simulink model "Practica1"  (R2025b)
settings: Solver=VariableStepAuto  StartTime=0.0  StopTime=200  RelTol=1e-3  AbsTol=1e-3
undefined symbols (not defined in the file): J, Km, L_a, R_a
libraries: fl_lib x13, nesl_utility x8
settings Model: Creator=chenfu  LastModifiedBy=chenfu
settings SolverCC: AutoScaleAbsTol=off  AlgebraicLoopSolver=TrustRegion  MaxZcPerStep=1.0
settings DebuggingCC: UnconnectedInputMsg=warning  UnconnectedOutputMsg=warning  UnconnectedLineMsg=warning  SymbolicDimsDataTypeCodeGenerationDiagnostic=none
settings ModelReferenceCC: EnableRefExpFcnMdlSchedulingChecks=on
settings SFSimCC: CustomCodeUndefinedFunction=UseInterfaceOnly
settings RTWCC: GPUComputeCapability=3.5  DLArmComputeVersion=19.05
settings SimscapeCC: SimscapeLogType=all  SimscapeLogSimulationStatistics=on  SimscapeLogDataHistory=10000.0

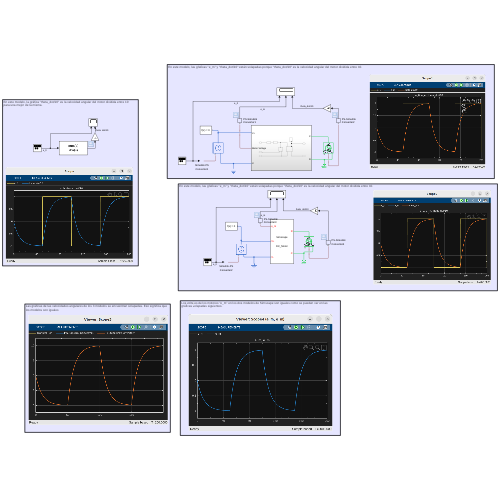
[thumbnail: Simulink's stored preview of the top-level diagram]
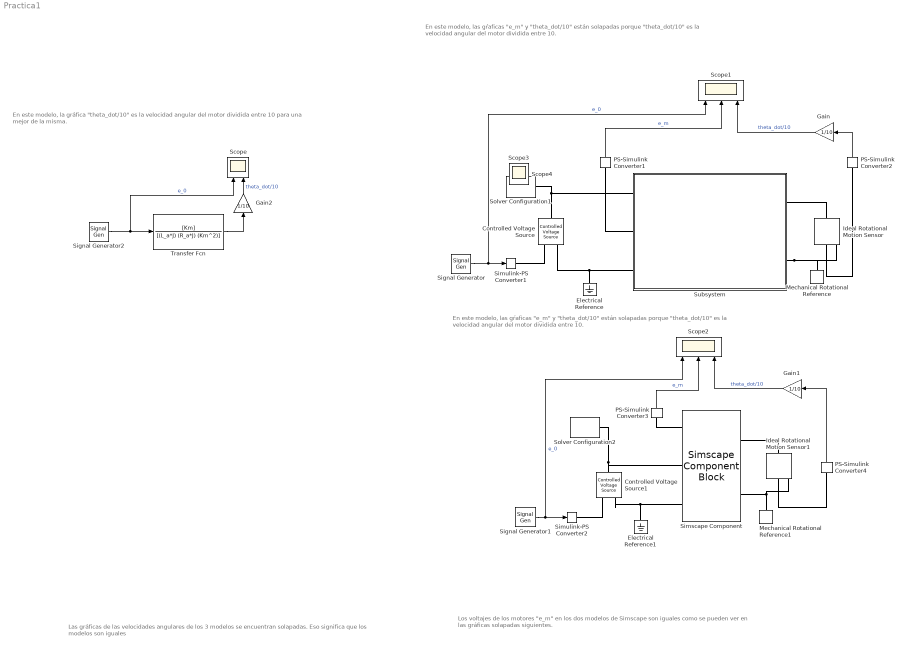
== system Practica1 ==
  note: En este modelo, la gráfica "theta_dot/10" es la velocidad angular del motor dividida entre 10
      | para una mejor de la misma.
  note: En este modelo, las gŕaficas "e_m" y "theta_dot/10" están solapadas porque "theta_dot/10" es la velocidad angular del motor dividida entre 10.
  note: En este modelo, las gŕaficas "e_m" y "theta_dot/10" están solapadas porque "theta_dot/10" es la velocidad angular del motor dividida entre 10.
  note: Los voltajes de los motores "e_m" en los dos modelos de Simscape son iguales como se pueden ver en las
      | gráficas solapadas siguientes.
  note: Las gráficas de las velocidades angulares de los 3 modelos se encuentran solapadas. Eso significa que
      | los modelos son iguales
  Controlled Voltage Source : fl_lib/Electrical/Electrical Sources/Controlled Voltage Source
  Controlled Voltage Source1 : fl_lib/Electrical/Electrical Sources/Controlled Voltage Source
  Electrical Reference : fl_lib/Electrical/Electrical Elements/Electrical Reference
  Electrical Reference1 : fl_lib/Electrical/Electrical Elements/Electrical Reference
  Gain : Gain  Gain=1/10
  Gain1 : Gain  Gain=1/10
  Gain2 : Gain  Gain=1/10
  Ideal Rotational Motion Sensor : fl_lib/Mechanical/Mechanical Sensors/Ideal Rotational Motion Sensor  reference=foundation.enum.MeasurementReference.difference  acceleration_port=false  velocity_port=true  position_port=true  wrap_angle=false  offset=0 rad
  Ideal Rotational Motion Sensor1 : fl_lib/Mechanical/Mechanical Sensors/Ideal Rotational Motion Sensor  reference=foundation.enum.MeasurementReference.difference  acceleration_port=false  velocity_port=true  position_port=true  wrap_angle=false  offset=0 rad
  Mechanical Rotational Reference : fl_lib/Mechanical/Rotational Elements/Mechanical Rotational Reference
  Mechanical Rotational Reference1 : fl_lib/Mechanical/Rotational Elements/Mechanical Rotational Reference
  PS-Simulink Converter{1..4} (4 alike) : nesl_utility/PS-Simulink Converter  PhysicalDomain=network_engine_domain  SubClassName=ps_output  LeftPortType=input  RightPortType=output  PseudoPeriodic=off  Frequencies=[]  VectorFormat=inherit  Unit=inherit  AffineConversion=off
  Scope : Scope  NumInputPorts=2
      settings: ActiveDisplayYMinimum=-1.25  ActiveDisplayYMaximum=1.25  DataLoggingVariableName=ScopeData2
  Scope1 : Scope  NumInputPorts=3
      settings: ActiveDisplayYMinimum=-1  ActiveDisplayYMaximum=1
  Scope2 : Scope  NumInputPorts=3
      settings: ActiveDisplayYMinimum=-1.25  ActiveDisplayYMaximum=1.25
  Signal Generator : SignalGenerator  WaveForm=square  Frequency=0.01
  Signal Generator1 : SignalGenerator  WaveForm=square  Frequency=0.01
  Signal Generator2 : SignalGenerator  WaveForm=square  Frequency=0.01
  Simscape Component : SimscapeComponentBlock  SourceFile=DC_Motor  ComponentPath=DC_Motor  ComponentVariants="[\"DC_Motor\"]"  ComponentVariantNames="[\"DC_Motor\"]"  ClassName=DC_Motor  SchemaVersion=1  res=10.0 Ohm  l=1e-2 H  J=1e-2 kg*m^2  bEMF=1e-1 V*s/rad  e_o_specify=off  e_o_priority=None  e_o=0 V  e_o_nominal_specify=off  e_o_nominal_value=1  e_o_nominal_unit=V  e_m_specify=off  e_m_priority=None  e_m=0 V  e_m_nominal_specify=off  e_m_nominal_value=1  e_m_nominal_unit=V  w_specify=off  w_priority=None  w=0 rad/s  w_nominal_specify=off  w_nominal_value=1  w_nominal_unit=rad/s  t_specify=off  t_priority=None  t=0 N*m  t_nominal_specify=off  t_nominal_value=1  t_nominal_unit=N*m  i_specify=off  i_priority=None  i=0 A  i_nominal_specify=off  i_nominal_value=1  i_nominal_unit=A
      settings: CopyFcn=simscape.sscblock.internal.componentBlockCallback(gcbh,'COPY')  PreCopyFcn=simscape.sscblock.internal.componentBlockCallback(gcbh,'PRECOPY')  PreDeleteFcn=simscape.sscblock.internal.componentBlockCallback(gcbh,'PREDELETE')  InternalSimscapePortConfiguration="{\"Bottom\":[],\"Left\":[{\"id\":\"V\",\"label\":\"e_m\",\"type\":\"output\"},{\"id\":\"vmas\",\"label\":\"V+\",\"type\":\"foundation.electrical.electrical\"},{\"id\":\"vmenos\",\"label\":\"V-\",\"type\":\"foundation.electrical.electrical\"}],\"Right\":[{\"id\":\"R\",\"label\":\"R\",\"type\":\"foundation.mechanical.rotational.rotational\"},{\"id\":\"C\",\"label\":\"C\",\"type\":\"foundation.mechanical.rotational.rotational\"}],\"Top\":[]}"
      mask Type: Simple Simscape component
  Simulink-PS Converter1 : nesl_utility/Simulink-PS Converter  PhysicalDomain=network_engine_domain  SubClassName=ps_input  LeftPortType=input  RightPortType=output  PseudoPeriodic=off  Frequencies=[]  NoiseDistribution=none  NoiseParameters=[]  Unit=1  AffineConversion=off  FilteringAndDerivatives=provide  SimscapeFilterOrder=1  InputFilterTimeConstant=0.001  UdotUserProvided=0
  Simulink-PS Converter2 : nesl_utility/Simulink-PS Converter  PhysicalDomain=network_engine_domain  SubClassName=ps_input  LeftPortType=input  RightPortType=output  PseudoPeriodic=off  Frequencies=[]  NoiseDistribution=none  NoiseParameters=[]  Unit=1  AffineConversion=off  FilteringAndDerivatives=filter  SimscapeFilterOrder=1  InputFilterTimeConstant=0.001  UdotUserProvided=0
  Solver Configuration1 : nesl_utility/Solver Configuration  PhysicalDomain=network_engine_domain  SubClassName=solver  LeftPortType=input  RightPortType=generic  Tones=[]  Harmonics=[]  SimulateNoise=off  Profile=off  UseLocalSampling=off  EnableSwitchedLinearOptims=on  FrequencyDomain=off  UseCCode=off  RelTol=0.001  AbsTol=0.001  MinStep=1e-09  ToWorkspace=off  RevertToSquareIcSolve=off  NumHomotopyIterations=100  PhasorMode=off  PhasorModeNumHarmonics=1  ConsistencySolver=NEWTON_XTOL_AFTER_FTOL  IndexReductionMethod=DerivativeReplacement  DoDC=off  ResidualTolerance=1e-09  ConsistencyTolSource=GLOBAL  ConsistencyAbsTol=0.001  ConsistencyRelTol=0.001  ConsistencyTolFactor=0.001  UseLocalSolver=off  LocalSolverChoice=NE_BACKWARD_EULER_ADVANCER  ResolveIndetEquations=on  FunctionEvalNumThread=1  LocalSolverSampleTime=0.001  DoFixedCost=off  MaxNonlinIter=3  MaxModeIter=2  ComputeImpulses=off  ImpulseIterations=2  LinearAlgebra=auto  LinearAlgebraNumThread=0  EquationFormulation=NE_TIME_EF  DelaysMemoryBudget=1024  AutomaticFiltering=on  FilteringTimeConstant=0.001  PartitionStorageMethod=AS_NEEDED  PartitionMemoryBudget=1024  PartitionMethod=ROBUST  MultibodyUseLocalSolver=off  MultibodyLocalSolverChoice=ODE1  MultibodyLocalSolverSampleTime=0.001
  Solver Configuration2 : nesl_utility/Solver Configuration  PhysicalDomain=network_engine_domain  SubClassName=solver  LeftPortType=input  RightPortType=generic  Tones=[]  Harmonics=[]  SimulateNoise=off  Profile=off  UseLocalSampling=off  EnableSwitchedLinearOptims=on  FrequencyDomain=off  UseCCode=off  RelTol=0.001  AbsTol=0.001  MinStep=1e-09  ToWorkspace=off  RevertToSquareIcSolve=off  NumHomotopyIterations=100  PhasorMode=off  PhasorModeNumHarmonics=1  ConsistencySolver=NEWTON_XTOL_AFTER_FTOL  IndexReductionMethod=DerivativeReplacement  DoDC=off  ResidualTolerance=1e-09  ConsistencyTolSource=GLOBAL  ConsistencyAbsTol=0.001  ConsistencyRelTol=0.001  ConsistencyTolFactor=0.001  UseLocalSolver=off  LocalSolverChoice=NE_BACKWARD_EULER_ADVANCER  ResolveIndetEquations=on  FunctionEvalNumThread=1  LocalSolverSampleTime=0.001  DoFixedCost=off  MaxNonlinIter=3  MaxModeIter=2  ComputeImpulses=off  ImpulseIterations=2  LinearAlgebra=auto  LinearAlgebraNumThread=0  EquationFormulation=NE_TIME_EF  DelaysMemoryBudget=1024  AutomaticFiltering=on  FilteringTimeConstant=0.001  PartitionStorageMethod=AS_NEEDED  PartitionMemoryBudget=1024  PartitionMethod=ROBUST  MultibodyUseLocalSolver=off  MultibodyLocalSolverChoice=ODE1  MultibodyLocalSolverSampleTime=0.001
  Subsystem : Subsystem
  Transfer Fcn : TransferFcn  Numerator=[Km]  Denominator=[(L_a*J) (R_a*J) (Km^2)]
  Scope3 : Scope
      settings: ActiveDisplayYMinimum=-12.405916089896222  ActiveDisplayYMaximum=12.338623681139223  DataLoggingVariableName=ScopeData3
  Scope4 : Scope
      settings: ActiveDisplayYMinimum=-1.2405916089222164  ActiveDisplayYMaximum=1.2338623675072702  DataLoggingVariableName=ScopeData4
  wires:
  Signal Generator/1 -> Scope1/1, Simulink-PS Converter1/1  "e_0"
  PS-Simulink Converter1/1 -> Scope1/2  "e_m"
  Gain/1 -> Scope1/3  "theta_dot/10"
  PS-Simulink Converter2/1 -> Gain/1
  Signal Generator1/1 -> Scope2/1, Simulink-PS Converter2/1  "e_0"
  PS-Simulink Converter4/1 -> Gain1/1
  PS-Simulink Converter3/1 -> Scope2/2  "e_m"
  Signal Generator2/1 -> Scope/1, Transfer Fcn/1  "e_0"
  Transfer Fcn/1 -> Gain2/1
  Gain2/1 -> Scope/2  "theta_dot/10"
  Gain1/1 -> Scope2/3  "theta_dot/10"
  connections:
  Controlled Voltage Source/LConn1 -- Solver Configuration1/RConn1 -- Subsystem/LConn1
  Controlled Voltage Source/RConn2 -- Electrical Reference/LConn1 -- Subsystem/LConn3
  Simulink-PS Converter1/RConn1 -- Controlled Voltage Source/RConn1
  Subsystem/RConn1 -- Ideal Rotational Motion Sensor/LConn1
  Subsystem/RConn2 -- Ideal Rotational Motion Sensor/RConn1 -- Mechanical Rotational Reference/LConn1
  Subsystem/LConn2 -- PS-Simulink Converter1/LConn1
  PS-Simulink Converter2/LConn1 -- Ideal Rotational Motion Sensor/RConn2
  Controlled Voltage Source1/RConn2 -- Simscape Component/LConn3 -- Electrical Reference1/LConn1
  Controlled Voltage Source1/LConn1 -- Solver Configuration2/RConn1 -- Simscape Component/LConn2
  Simulink-PS Converter2/RConn1 -- Controlled Voltage Source1/RConn1
  Mechanical Rotational Reference1/LConn1 -- Ideal Rotational Motion Sensor1/RConn1 -- Simscape Component/RConn2
  Ideal Rotational Motion Sensor1/RConn2 -- PS-Simulink Converter4/LConn1
  Simscape Component/RConn1 -- Ideal Rotational Motion Sensor1/LConn1
  PS-Simulink Converter3/LConn1 -- Simscape Component/LConn1

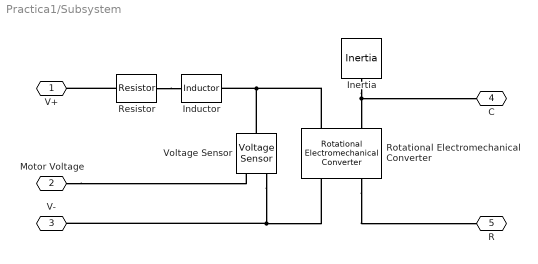
== system Practica1/Subsystem ==
  Inductor : fl_lib/Electrical/Electrical Elements/Inductor  l=10 mH  r=0 Ohm  g=0 1/Ohm  i_specify=off  i_priority=None  i=0 A  i_nominal_specify=off  i_nominal_value=1  i_nominal_unit=A  v_specify=off  v_priority=None  v=0 V  v_nominal_specify=off  v_nominal_value=1  v_nominal_unit=V  i_L_specify=off  i_L_priority=High  i_L=0 A  i_L_nominal_specify=off  i_L_nominal_value=1  i_L_nominal_unit=A
  Inertia : fl_lib/Mechanical/Rotational Elements/Inertia  inertia=0.01 kg*m^2  num_ports=foundation.enum.numPorts2.one  w_specify=off  w_priority=High  w=0 rad/s  w_nominal_specify=off  w_nominal_value=1  w_nominal_unit=rad/s  t_specify=off  t_priority=None  t=0 N*m  t_nominal_specify=off  t_nominal_value=1  t_nominal_unit=N*m
  Resistor : fl_lib/Electrical/Electrical Elements/Resistor  R=10 Ohm  i_specify=off  i_priority=None  i=0 A  i_nominal_specify=off  i_nominal_value=1  i_nominal_unit=A  v_specify=off  v_priority=None  v=0 V  v_nominal_specify=off  v_nominal_value=1  v_nominal_unit=V
  Rotational Electromechanical Converter : fl_lib/Electrical/Electrical Elements/Rotational Electromechanical Converter  K=0.1 V*s/rad  i_specify=off  i_priority=None  i=0 A  i_nominal_specify=off  i_nominal_value=1  i_nominal_unit=A  v_specify=off  v_priority=None  v=0 V  v_nominal_specify=off  v_nominal_value=1  v_nominal_unit=V  t_specify=off  t_priority=None  t=0 N*m  t_nominal_specify=off  t_nominal_value=1  t_nominal_unit=N*m  w_specify=off  w_priority=None  w=0 rad/s  w_nominal_specify=off  w_nominal_value=1  w_nominal_unit=rad/s
  Voltage Sensor : fl_lib/Electrical/Electrical Sensors/Voltage Sensor
  V+ : PMIOPort  Side=Left
  Motor Voltage : PMIOPort  Port=2  Side=Left
  V- : PMIOPort  Port=3  Side=Left
  C : PMIOPort  Port=4  Side=Right
  R : PMIOPort  Port=5  Side=Right
  connections:
  Resistor/RConn1 -- Inductor/LConn1
  Rotational Electromechanical Converter/RConn2 -- R/RConn1
  Inertia/LConn1 -- Rotational Electromechanical Converter/LConn2 -- C/RConn1
  Resistor/LConn1 -- V+/RConn1
  Rotational Electromechanical Converter/LConn1 -- Inductor/RConn1 -- Voltage Sensor/LConn1
  Voltage Sensor/RConn2 -- Rotational Electromechanical Converter/RConn1 -- V-/RConn1
  Motor Voltage/RConn1 -- Voltage Sensor/RConn1
